simulink model "ME4564_Project2"  (R2021a)
settings: Solver=VariableStepAuto  StartTime=0.0  StopTime=15  RelTol=1e-3
libraries: slpidlib x1
settings Model: Creator=Sam Kramer  LastModifiedBy=Sam Kramer

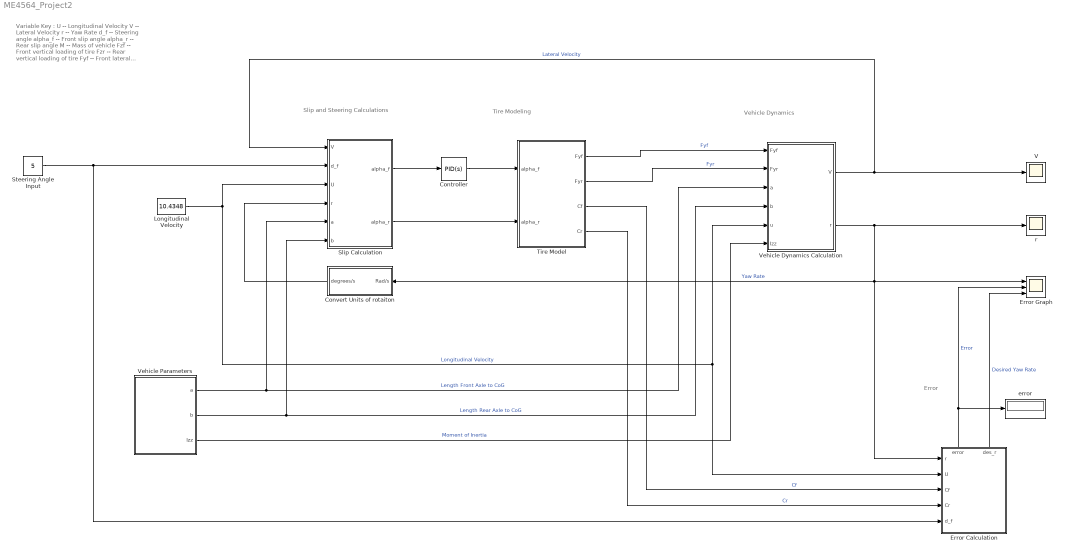
== system ME4564_Project2 ==
  note: Error
  note: Vehicle Dynamics
  note: Tire Modeling
  note: Slip and Steering Calculations
  note: Variable Key :
      | U -- Longitudinal Velocity
      | V -- Lateral Velocity
      | r -- Yaw Rate
      | d_f -- Steering angle
      | alpha_f -- Front slip angle
      | alpha_r -- Rear slip angle
      | M -- Mass of vehicle
      | Fzf -- Front vertical loading of tire
      | Fzr -- Rear vertical loading of tire
      | Fyf -- Front lateral loading of tire
      | Fyr -- Rear lateral loading of tire
      | Cf -- Front cornering stiffness
      | Cr -- Rear cornering stiffness
      | e -- yaw rate error
  Controller : slpidlib/PID Controller  Controller=PID  Form=Parallel  TimeDomain=Continuous-time  UseExternalTs=off  SampleTime=-1  IntegratorMethod=Forward Euler  FilterMethod=Forward Euler  ControllerParametersSource=internal  P=-7  I=100  D=100  UseFilter=on  N=50  TunerSelectOption=Transfer Function Based (PID Tuner App)  InitialConditionSource=internal  InitialConditionForIntegrator=0  InitialConditionForFilter=0  DifferentiatorICPrevScaledInput=0  ExternalReset=none  TrackingMode=off  Kt=1  LimitOutput=off  SatLimitsSource=internal  UpperSaturationLimit=inf  LowerSaturationLimit=-inf  LinearizeAsGain=on  AntiWindupMode=none  Kb=1  POutMin=[]  POutMax=[]  IOutMin=[]  IOutMax=[]  DOutMin=[]  DOutMax=[]  NOutMin=[]  NOutMax=[]  SumOutMin=[]  SumOutMax=[]  SaturationOutMin=[]  SaturationOutMax=[]  PParamMin=[]  PParamMax=[]  IParamMin=[]  IParamMax=[]  DParamMin=[]  DParamMax=[]  NParamMin=[]  NParamMax=[]  KbParamMin=[]  KbParamMax=[]  KtParamMin=[]  KtParamMax=[]  KbOutMin=[]  KbOutMax=[]  KtOutMin=[]  KtOutMax=[]  IntegratorOutMin=[]  IntegratorOutMax=[]  FilterOutMin=[]  FilterOutMax=[]  SumI1OutMin=[]  SumI1OutMax=[]  SumI2OutMin=[]  SumI2OutMax=[]  SumI3OutMin=[]  SumI3OutMax=[]  SumI4OutMin=[]  SumI4OutMax=[]  SumDOutMin=[]  SumDOutMax=[]  DifferentiatorOutMin=[]  DifferentiatorOutMax=[]  FilterDiffOutCoefMin=[]  FilterDiffOutCoefMax=[]  ReciprocalOutMin=[]  ReciprocalOutMax=[]  SumDenOutMin=[]  SumDenOutMax=[]  SumNumOutMin=[]  SumNumOutMax=[]  DivideOutMin=[]  DivideOutMax=[]  UdiffTsProdOutMin=[]  UdiffTsProdOutMax=[]  NTsProdOutMin=[]  NTsProdOutMax=[]  UintegralTsProdOutMin=[]  UintegralTsProdOutMax=[]  UngainTsProdOutMin=[]  UngainTsProdOutMax=[]  IntegratorContinuousStateAttributes=''  IntegratorStateMustResolveToSignalObject=off  IntegratorRTWStateStorageClass=Auto  FilterContinuousStateAttributes=''  FilterStateMustResolveToSignalObject=off  FilterRTWStateStorageClass=Auto  ParallelPVariant=InternalParameters  IdealPVariant=Disabled  IVariant=InternalParameters  DVariant=InternalParameters  IntegratorVariant=Continuous  SatVariant=Disabled  AWVariant=Passthrough  PCopyVariant=Disabled  TRVariant=Disabled  FdbkBlocksVariant=Forward  IdealPFdbkVariant=Disabled  SatFdbkVariant=Disabled  DerivativeFilterVariant=ContFilter  NVariant=InternalParameters  NCopyVariant=Disabled  FilterICVariant=InternalICsFilter  IntegratorICVariant=InternalICs  ExternalResetVariant=Disabled  TRSumVariant=Passthrough  SumFdbkVariant=Disabled  SumVariant=Sum_PID  TsampFilterVariant=InternalTs  TsampNgainVariant=Passthrough  TsampIntegralVariant=Passthrough  ExternalSaturationOutDataTypeStr=Inherit: Same as second input
  Convert Units of rotaiton : Subsystem
  Error Calculation : Subsystem
      settings: PortSchema="{\"entries\":[{\"content\":{\"sides\":[{\"content\":{\"connectorIds\":[\"In1\",\"In2\",\"In3\",\"In4\",\"In5\"]},\"type\":\"ConnectorPlacement.EquallySpacedRectSide\",\"uuid\":\"a37d6160-6c55-497b-b36e-de5448ed4b4d\"},{\"content\":{\"connectorIds\":[],\"side\":\"RIGHT\"},\"type\":\"ConnectorPlacement.EquallySpacedRectSide\",\"uuid\":\"39052553-47e2-4383-a9bb-c293271c24fb\"},{\"content\":{\"connectorIds\":[\"Out1\",\"Out2\"],\"side\":\"TOP\"},\"type\":\"ConnectorPlacement.EquallySpacedRectSide\",\"uuid\":\"477127ec-445c-4e01-81a8-e59f976cceef\"}]},\"type\":\"ConnectorPlacement.EquallySpacedConnector\",\"uuid\":\"512eb71f-2657-44f4-9c5d-78553267f42c\"}],\"packageUris\":[\"http://schema.mathworks.com/mf0/Connector/R2020b\"],\"version\":\"1.0\"}"
  Error Graph : Scope  NumInputPorts=3
  Longitudinal Velocity : Constant  Value=10.4348
  Slip Calculation : Subsystem
  Steering Angle Input : Constant  Value=5
  Tire Model : Subsystem
  V : Scope
  Vehicle Dynamics Calculation : Subsystem
  Vehicle Parameters : Subsystem
  error : Display
  r : Scope
  wires:
  Steering Angle Input/1 -> Error Calculation/5(d_f), Slip Calculation/2(d_f)
  Longitudinal Velocity/1 -> Vehicle Dynamics Calculation/5(u), Error Calculation/2(U), Slip Calculation/3(U)  "Longitudinal Velocity"
  Tire Model/2(Fyr) -> Vehicle Dynamics Calculation/2(Fyr)  "Fyr"
  Tire Model/1(Fyf) -> Vehicle Dynamics Calculation/1(Fyf)  "Fyf"
  Vehicle Dynamics Calculation/1(V) -> Slip Calculation/1(V), V/1  "Lateral Velocity"
  Vehicle Dynamics Calculation/2(r) -> r/1, Error Calculation/1(r), Error Graph/1, Convert Units of rotaiton/1(Rad/s)  "Yaw Rate"
  Vehicle Parameters/1(a) -> Vehicle Dynamics Calculation/3(a), Slip Calculation/5(a)  "Length Front Axle to CoG"
  Vehicle Parameters/3(Izz) -> Vehicle Dynamics Calculation/6(Izz)  "Moment of Inertia"
  Vehicle Parameters/2(b) -> Vehicle Dynamics Calculation/4(b), Slip Calculation/6(b)  "Length Rear Axle to CoG"
  Tire Model/3(Cf) -> Error Calculation/3(Cf)  "Cf"
  Tire Model/4(Cr) -> Error Calculation/4(Cr)  "Cr"
  Error Calculation/1(error) -> Error Graph/2, error/1  "Error"
  Error Calculation/2(des_r) -> Error Graph/3  "Desired Yaw Rate"
  Slip Calculation/1(alpha_f) -> Controller/1
  Convert Units of rotaiton/1(degrees/s) -> Slip Calculation/4(r)
  Slip Calculation/2(alpha_r) -> Tire Model/2(alpha_r)
  Controller/1 -> Tire Model/1(alpha_f)

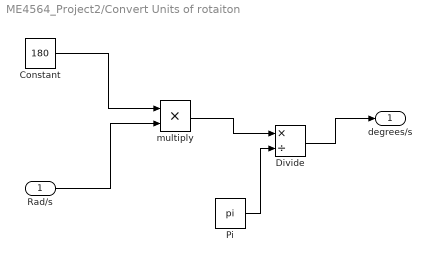
== system ME4564_Project2/Convert Units of rotaiton ==
  Rad/s : Inport
  Constant : Constant  Value=180
  Divide : Product  Inputs=*/
  Pi : Constant  Value=pi  OutDataTypeStr=Inherit: Inherit via back propagation
  multiply : Product
  degrees/s : Outport
  wires:
  Rad/s/1 -> multiply/2
  Constant/1 -> multiply/1
  Pi/1 -> Divide/2
  multiply/1 -> Divide/1
  Divide/1 -> degrees/s/1

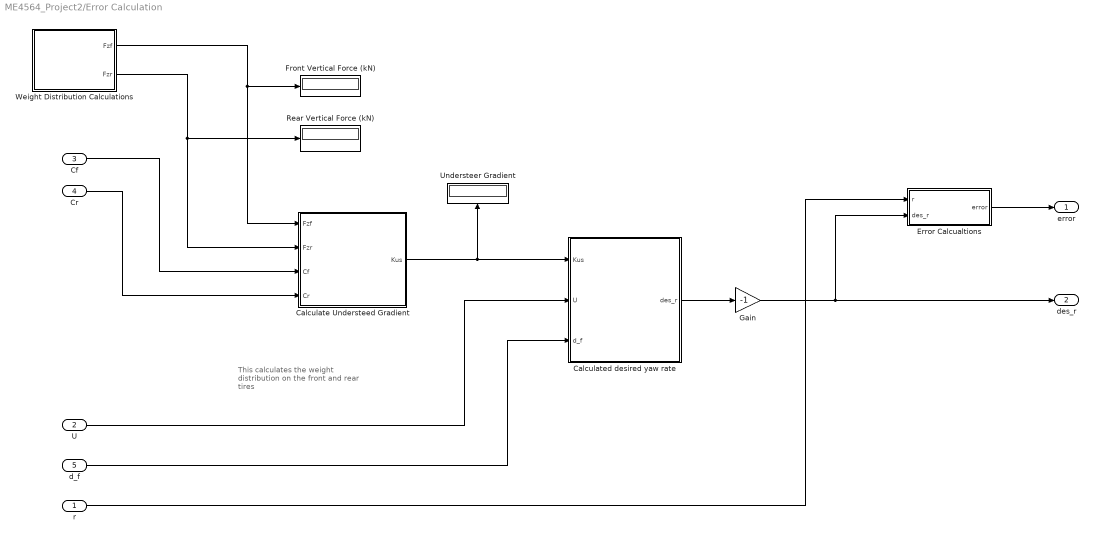
== system ME4564_Project2/Error Calculation ==
  note: This calculates the weight distribution on the front and rear tires
  r : Inport
  U : Inport  Port=2
  Cf : Inport  Port=3
  Cr : Inport  Port=4
  d_f : Inport  Port=5
  Calculate Understeed Gradient : MATLAB Function  TreatAsAtomicUnit=on
  Calculated desired yaw rate : MATLAB Function  TreatAsAtomicUnit=on
  Error Calcualtions : Subsystem
  Front Vertical Force (kN) : Display
      settings: Decimation=3
  Gain : Gain  Gain=-1
  Rear Vertical Force (kN) : Display
  Understeer Gradient : Display
      settings: Decimation=3
  Weight Distribution Calculations : Subsystem
  error : Outport
  des_r : Outport  Port=2
  wires:
  Weight Distribution Calculations/2(Fzr) -> Calculate Understeed Gradient/2(Fzr), Rear Vertical Force (kN)/1
  Weight Distribution Calculations/1(Fzf) -> Calculate Understeed Gradient/1(Fzf), Front Vertical Force (kN)/1
  Cf/1 -> Calculate Understeed Gradient/3(Cf)
  Cr/1 -> Calculate Understeed Gradient/4(Cr)
  Calculate Understeed Gradient/1(Kus) -> Understeer Gradient/1, Calculated desired yaw rate/1(Kus)
  r/1 -> Error Calcualtions/1(r)
  U/1 -> Calculated desired yaw rate/2(U)
  d_f/1 -> Calculated desired yaw rate/3(d_f)
  Calculated desired yaw rate/1(des_r) -> Gain/1
  Error Calcualtions/1(error) -> error/1
  Gain/1 -> des_r/1, Error Calcualtions/2(des_r)

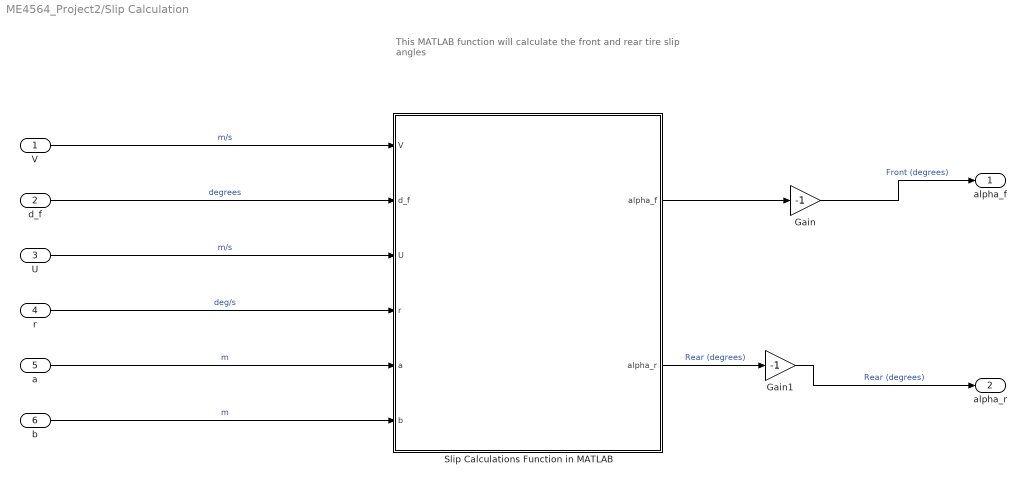
== system ME4564_Project2/Slip Calculation ==
  note: This MATLAB function will calculate the front and rear tire slip angles
  V : Inport
  d_f : Inport  Port=2
  U : Inport  Port=3
  r : Inport  Port=4
  a : Inport  Port=5
  b : Inport  Port=6
  Gain : Gain  Gain=-1
  Gain1 : Gain  Gain=-1
  Slip Calculations Function in MATLAB : MATLAB Function  TreatAsAtomicUnit=on
  alpha_f : Outport
  alpha_r : Outport  Port=2
  wires:
  V/1 -> Slip Calculations Function in MATLAB/1(V)  "m/s"
  d_f/1 -> Slip Calculations Function in MATLAB/2(d_f)  "degrees"
  U/1 -> Slip Calculations Function in MATLAB/3(U)  "m/s"
  r/1 -> Slip Calculations Function in MATLAB/4(r)  "deg/s"
  Slip Calculations Function in MATLAB/1(alpha_f) -> Gain/1
  Slip Calculations Function in MATLAB/2(alpha_r) -> Gain1/1  "Rear (degrees)"
  a/1 -> Slip Calculations Function in MATLAB/5(a)  "m"
  b/1 -> Slip Calculations Function in MATLAB/6(b)  "m"
  Gain/1 -> alpha_f/1  "Front (degrees)"
  Gain1/1 -> alpha_r/1  "Rear (degrees)"

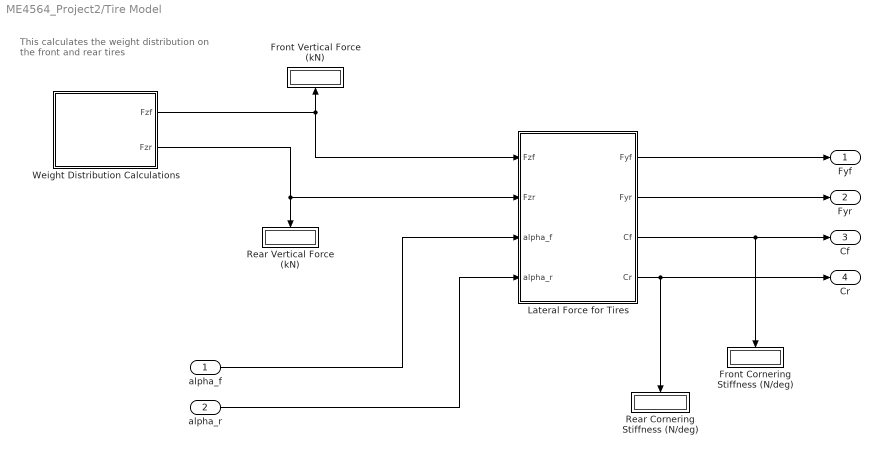
== system ME4564_Project2/Tire Model ==
  note: This calculates the weight
      | distribution on the front and rear
      | tires
  alpha_f : Inport
  alpha_r : Inport  Port=2
  Front Cornering Stiffness (N/deg) : Display
  Front Vertical Force (kN) : Display
      settings: Decimation=3
  Lateral Force for Tires : MATLAB Function  TreatAsAtomicUnit=on
  Rear Cornering Stiffness (N/deg) : Display
  Rear Vertical Force (kN) : Display
  Weight Distribution Calculations : Subsystem
  Fyf : Outport
  Fyr : Outport  Port=2
  Cf : Outport  Port=3
  Cr : Outport  Port=4
  wires:
  Weight Distribution Calculations/1(Fzf) -> Lateral Force for Tires/1(Fzf), Front Vertical Force (kN)/1
  Weight Distribution Calculations/2(Fzr) -> Lateral Force for Tires/2(Fzr), Rear Vertical Force (kN)/1
  Lateral Force for Tires/4(Cr) -> Cr/1, Rear Cornering Stiffness (N/deg)/1
  Lateral Force for Tires/3(Cf) -> Cf/1, Front Cornering Stiffness (N/deg)/1
  alpha_f/1 -> Lateral Force for Tires/3(alpha_f)
  Lateral Force for Tires/1(Fyf) -> Fyf/1
  alpha_r/1 -> Lateral Force for Tires/4(alpha_r)
  Lateral Force for Tires/2(Fyr) -> Fyr/1

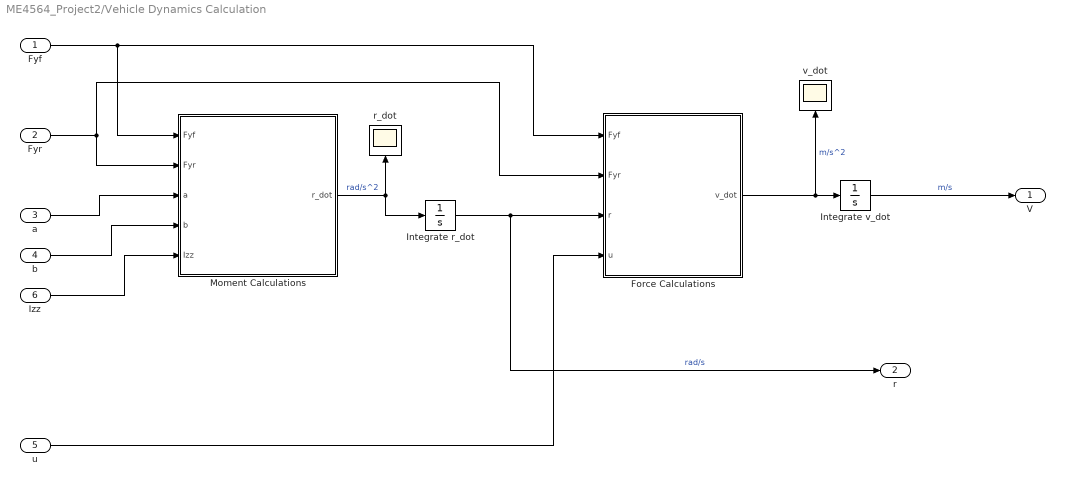
== system ME4564_Project2/Vehicle Dynamics Calculation ==
  Fyf : Inport
  Fyr : Inport  Port=2
  a : Inport  Port=3
  b : Inport  Port=4
  u : Inport  Port=5
  Izz : Inport  Port=6
  Force Calculations : MATLAB Function  TreatAsAtomicUnit=on
  Integrate r_dot : Integrator
  Integrate v_dot : Integrator
  Moment Calculations : MATLAB Function  TreatAsAtomicUnit=on
  r_dot : Scope
  v_dot : Scope
  V : Outport
  r : Outport  Port=2
  wires:
  Fyf/1 -> Force Calculations/1(Fyf), Moment Calculations/1(Fyf)
  Fyr/1 -> Force Calculations/2(Fyr), Moment Calculations/2(Fyr)
  a/1 -> Moment Calculations/3(a)
  b/1 -> Moment Calculations/4(b)
  Izz/1 -> Moment Calculations/5(Izz)
  Moment Calculations/1(r_dot) -> Integrate r_dot/1, r_dot/1  "rad/s^2"
  Integrate r_dot/1 -> Force Calculations/3(r), r/1  "rad/s"
  u/1 -> Force Calculations/4(u)
  Force Calculations/1(v_dot) -> v_dot/1, Integrate v_dot/1  "m/s^2"
  Integrate v_dot/1 -> V/1  "m/s"

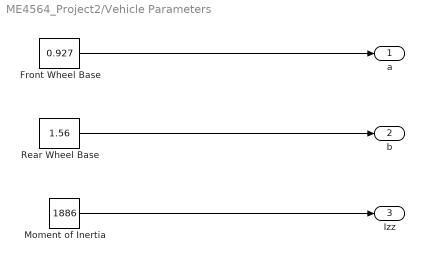
== system ME4564_Project2/Vehicle Parameters ==
  Front Wheel Base : Constant  Value=0.927
  Moment of Inertia : Constant  Value=1886
  Rear Wheel Base : Constant  Value=1.56
  a : Outport
  b : Outport  Port=2
  Izz : Outport  Port=3
  wires:
  Front Wheel Base/1 -> a/1
  Rear Wheel Base/1 -> b/1
  Moment of Inertia/1 -> Izz/1

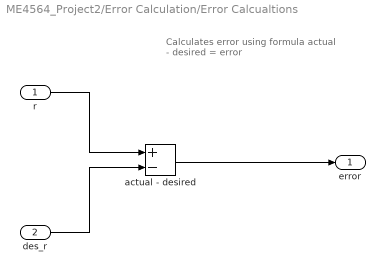
== system ME4564_Project2/Error Calculation/Error Calcualtions ==
  note: Calculates error using formula
      |
      | actual - desired = error
  r : Inport
  des_r : Inport  Port=2
  " actual - desired" : Sum  Inputs=+-
  error : Outport
  wires:
  " actual - desired"/1 -> error/1
  r/1 -> " actual - desired"/1
  des_r/1 -> " actual - desired"/2

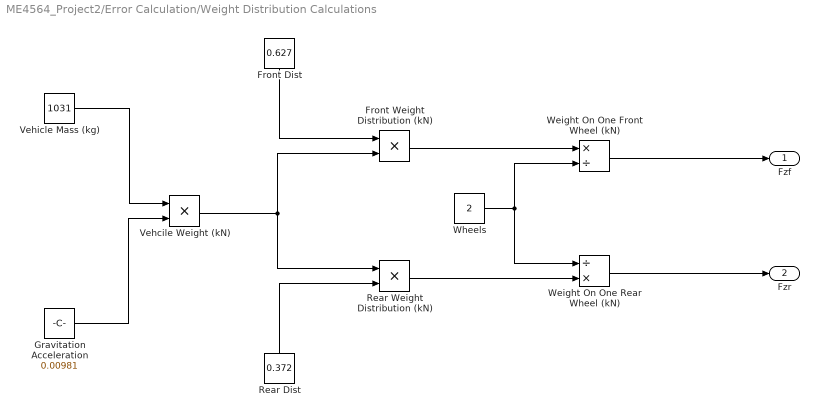
== system ME4564_Project2/Error Calculation/Weight Distribution Calculations ==
  Front Dist : Constant  Value=0.627
  Front Weight Distribution (kN) : Product
  Gravitation Acceleration : Constant  Value=0.00981
  Rear Dist : Constant  Value=0.372
  Rear Weight Distribution (kN) : Product
  Vehcile Weight (kN) : Product
  Vehicle Mass (kg) : Constant  Value=1031
  Weight On One Front Wheel (kN) : Product  Inputs=*/
  Weight On One Rear Wheel (kN) : Product  Inputs=/*
  Wheels : Constant  Value=2
  Fzf : Outport
  Fzr : Outport  Port=2
  wires:
  Vehicle Mass (kg)/1 -> Vehcile Weight (kN)/1
  Gravitation Acceleration/1 -> Vehcile Weight (kN)/2
  Vehcile Weight (kN)/1 -> Rear Weight Distribution (kN)/1, Front Weight Distribution (kN)/2
  Front Dist/1 -> Front Weight Distribution (kN)/1
  Wheels/1 -> Weight On One Front Wheel (kN)/2, Weight On One Rear Wheel (kN)/1
  Rear Dist/1 -> Rear Weight Distribution (kN)/2
  Rear Weight Distribution (kN)/1 -> Weight On One Rear Wheel (kN)/2
  Front Weight Distribution (kN)/1 -> Weight On One Front Wheel (kN)/1
  Weight On One Front Wheel (kN)/1 -> Fzf/1
  Weight On One Rear Wheel (kN)/1 -> Fzr/1

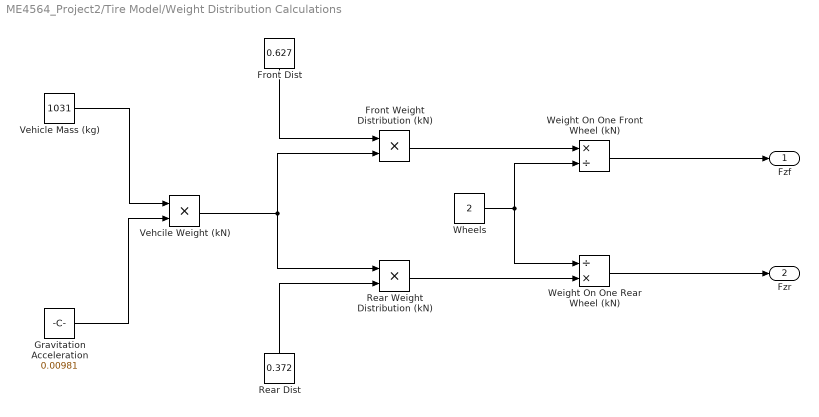
== system ME4564_Project2/Tire Model/Weight Distribution Calculations ==
  Front Dist : Constant  Value=0.627
  Front Weight Distribution (kN) : Product
  Gravitation Acceleration : Constant  Value=0.00981
  Rear Dist : Constant  Value=0.372
  Rear Weight Distribution (kN) : Product
  Vehcile Weight (kN) : Product
  Vehicle Mass (kg) : Constant  Value=1031
  Weight On One Front Wheel (kN) : Product  Inputs=*/
  Weight On One Rear Wheel (kN) : Product  Inputs=/*
  Wheels : Constant  Value=2
  Fzf : Outport
  Fzr : Outport  Port=2
  wires:
  Vehicle Mass (kg)/1 -> Vehcile Weight (kN)/1
  Gravitation Acceleration/1 -> Vehcile Weight (kN)/2
  Vehcile Weight (kN)/1 -> Rear Weight Distribution (kN)/1, Front Weight Distribution (kN)/2
  Front Dist/1 -> Front Weight Distribution (kN)/1
  Wheels/1 -> Weight On One Front Wheel (kN)/2, Weight On One Rear Wheel (kN)/1
  Rear Dist/1 -> Rear Weight Distribution (kN)/2
  Rear Weight Distribution (kN)/1 -> Weight On One Rear Wheel (kN)/2
  Front Weight Distribution (kN)/1 -> Weight On One Front Wheel (kN)/1
  Weight On One Front Wheel (kN)/1 -> Fzf/1
  Weight On One Rear Wheel (kN)/1 -> Fzr/1

== matlab function ME4564_Project2/Tire Model/Lateral Force for Tires ==
  data: Fzf input; Fyf output; Fzr input; alpha_f input; alpha_r input; Fyr output; Cf output; Cr output
function [Fyf,Fyr, Cf, Cr] = fcn(Fzf, Fzr, alpha_f, alpha_r)
%{
    This function will be used to calculate the lateral force for both the
    front and the rear tires. This will then be used to calculate the
    lateral velocity and the roll rate of the vehicle. The pacejka
    coefficients are calculated out of the loop so that they do not need to
    be repeated each cycle. The Pacejka Coefficients are hard coded because
    there are issues loading in the data using simulink.
    Sam Kramer                                                      22NOV22
%}

    % --Front tire lateral force
    
        % --Calculating Shy
            shf = (0.00688)*Fzf - 0.104585;
        
        % --Calculating alphay
            alphay = alpha_f + shf;
        
        % --Calculating C
            C = 1.457787;
        
        % --Calculating D
            Df = ((-15.6725)*(Fzf^2)) + ((-1022.181)*(Fzf));
        
        % --Calculating E
            Ef = (0.06087)*(Fzf) + (0.7014)*(1 - (-.1556))*sign(alphay);
        
        % --Calculating K
            Kf = (-1949)*sin(2*atan(Fzf / (-8.3265)));
        
        % --Calculating B
            Bf = Kf / (C*Df);
        
        % --Calculating Svy
            Svf = (-14.6492)*(Fzf) + (-75.3516);
            
        % --Calculate Ba (Slip angle composite)
            Baf = Bf*(alphay);
        
        % --Calculating Fyf
            Fyf = Df*sin(C*atan(Baf - Ef*(Baf - atan(Baf)))) + Svf;
            
        % --Define cornering stiffness
            Cf = Kf;         % Define cornering stiffness for front tire
    
    % --Rear tire lateral force
    
        % --Calculating Shy
            shr = (0.00688)*Fzr + (-0.10458);
        
        % --Calculating alphay
            alphayr = alpha_r + shr;
        
        % --Calculating D
            Dr = (-15.6725)*Fzr^2 + (-1022.2)*Fzr;
        
        % --Calculating E
            Er = (0.0609)*Fzr + (0.7014)*(1 - (-.1556)) * sign(alphayr);
        
        % --Calculating K
            Kr = (-1949)*sin(2*atan(Fzr/(-8.3265)));
        
        % --Calculating B
            Br = Kr/(C*Dr);
        
        % --Calculating Svy
            Svr = (-14.6492)*Fzr + (-75.3516);
            
        % --Calculating Bar
            Bar = Br * alphayr;
        
        % --Calculating Fyf
            Fyr = Dr*sin(C*atan(Bar - Er*(Bar - atan(Bar)))) + Svr;
            
        % --Calculating rear cornering stiffness
            Cr = Kr;         % Define cornering stiffness for rear tire

end

== matlab function ME4564_Project2/Slip Calculation/Slip Calculations Function in MATLAB ==
  data: V input; alpha_f output; d_f input; U input; r input; a input; b input; alpha_r output
function [alpha_f,alpha_r] = Slip_Calculations(V, d_f, U, r, a, b)
%{ 
    This will be the calculation of the slip angles for project two block
    number 1 within simulink. This will return two slip angles for the 
    front and rear tires.
            
        V = lateral velocity (m/s)
        d_f = steering angle (degrees)
        U = longitudinal velocity (m/s)
        r = yaw rate (rad/s)
        a = front wheel base (m)
        b = rear wheel base (m)

    Sam Kramer                                                      16NOV22
%}
    
    % --Front tire calculations
        alpha_f = d_f - (V + a*r)/U;      % Calculate front tire slip angle

    % --Rear tire calculations
        alpha_r = (V - b*r)/U;           % Calculate rear tire slip angle

end

== matlab function ME4564_Project2/Vehicle Dynamics Calculation/Moment Calculations ==
  data: Fyf input; r_dot output; Fyr input; a input; b input; Izz input
function r_dot = Moment_Equations(Fyf, Fyr, a, b, Izz)
%{
    This function will be used to calculate the yaw acceleration of the
    vehicle using the sum of moments equation. The yaw acceleration will be
    output and then an integrator block will be used to calculate the yaw
    velocity.

                        r' = (aFyf - bFyr)/Izz
            r' = yaw acceleration (rad/s^2)
            a = front wheel base (m)
            Fy = lateral force (N)
            b = rear wheel base (m)
            Izz = Mass moment of inertia (kg-m^2)

    Sam Kramer                                                      23NOV22

%}

    % --Calculate r_dot
        r_dot = (a*Fyf - b*Fyr)/Izz;        % Calcualte yaw acc (rad/s^2)

end

== matlab function ME4564_Project2/Vehicle Dynamics Calculation/Force Calculations ==
  data: Fyf input; Fyr input; r input; u input; v_dot output
function v_dot = Forces_Calculation(Fyf, Fyr, r, u)
%{ 
    This function will be used to calculate the lateral acceleration of the
    vehicle. This function will use sum of forces on the vehicle to
    calculate v_dot. An integrator will be used after to make the
    acceleration into the lateral velocity. This will follow the equation:
                        
                            v' = (Fy/M) - U*r
            r = yaw rate (rad/s)
            Fy = Lateral force (N)
            M = vehicle mass  (kg)
            U = longitudinal velocity (m/s)
            v' = lateral acceleration (m/s^2)

    Sam Kramer                                                      23NOV22

%}
    % --Parameters
        M = 1031;       % Mass of vehicle (kg)
 
    % --Calculate v_dot
        v_dot = ((Fyf + Fyr)/M) - u*r;
    

end

== matlab function ME4564_Project2/Error Calculation/Calculate Understeed Gradient ==
  data: Fzf input; Fzr input; Cf input; Kus output; Cr input
function Kus = Understeer(Fzf, Fzr, Cf, Cr)
%{
    This will be used to calcualte the understeer gradient for the use in
    the calculation of the desired yaw rate. This will be using the
    understeer gradient formula from the notes
    Sam Kramer                                                      29NOV22
%}

    % --Calculating Kus
        Kus = (Fzf/Cf) - (Fzr/Cr);
        
end

== matlab function ME4564_Project2/Error Calculation/Calculated desired yaw rate ==
  data: Kus input; des_r output; U input; d_f input
function des_r = desiredSteering(Kus, U, d_f)
%{
    This will be used to calculate the desired yaw rate that will be
    calculated off of the steering angle input.
    Sam Kramer                                                      29NOV22
%}

    % --Parameters
        L = 2.487;          % length of the vehicle (m)
        g = 9.81;           % gravitational constant (m/s^2)
        
    % --Calculate desired rate
        des_r = (U*d_f)/(L + Kus*(U^2/g));      % Desired yaw rate
        
    % --Convert to rad/s
        des_r = des_r * (3.1415 / 180);         % Desired yaw in rad/s
        
end
